simulink model "pruebas_filtro_lcl"  (R2024a)
settings: Solver=VariableStepAuto  StartTime=0.0  StopTime=5  RelTol=1e-3
libraries: spsThreePhaseSeriesRLCBranchLib x3, spsGroundLib x2, spsDCVoltageSourceLib x1, spsTwoLevelConverterLib x1, spsSVPWMGenerator2LevelLib x1, spsThreePhaseVIMeasurementLib x1, spsThreePhaseProgrammableVoltageSourceLib x1, sps_lib x1
settings Model: SimulationMode=accelerator  Creator=sebar  LastModifiedBy=sebar

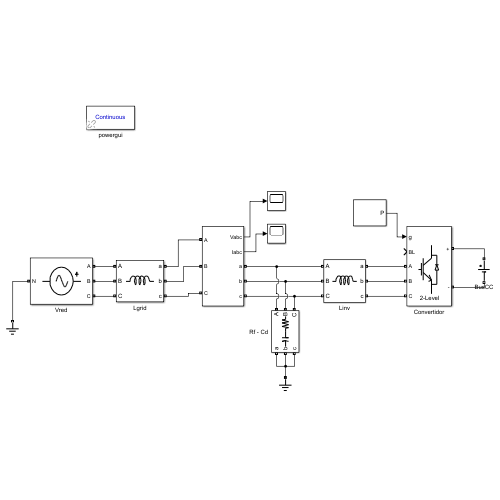
[thumbnail: Simulink's stored preview of the top-level diagram]
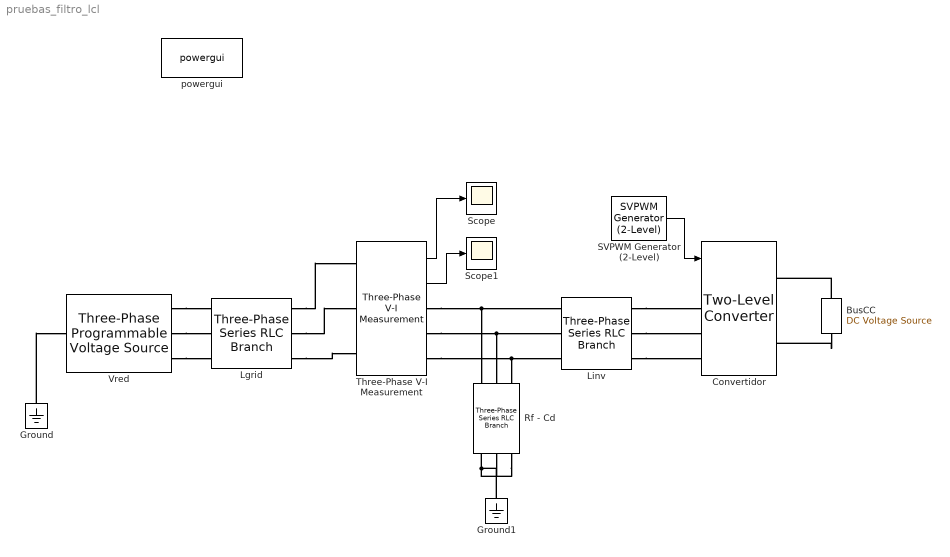
== system pruebas_filtro_lcl ==
  BusCC : spsDCVoltageSourceLib/DC Voltage Source  Amplitude=400  Measurements=None
  Convertidor : spsTwoLevelConverterLib/Two-Level Converter  ModelType=Switching devices  Ron=1e-3  Rs=1e6  Cs=inf  Vforward=[0,0]  Ron_Diode=1e-3  Rs_Diode=1e6  Cs_Diode=inf  Vf_Diode=1e-3  Rs_CurrentSource=inf  Ron_ACsource=1e-3
      settings: LibrarySourceBlock=sps_lib/Power Electronics/Two-Level Converter
  Ground : spsGroundLib/Ground  LConnTagsString=a
  Ground1 : spsGroundLib/Ground  LConnTagsString=a
  Lgrid : spsThreePhaseSeriesRLCBranchLib/Three-Phase Series RLC Branch  LConnTagsString=A|B|C  RConnTagsString=A|B|C  BranchType=L  Resistance=1  Inductance=273e-6  Capacitance=1e-6  Measurements=None
  Linv : spsThreePhaseSeriesRLCBranchLib/Three-Phase Series RLC Branch  LConnTagsString=A|B|C  RConnTagsString=A|B|C  BranchType=L  Resistance=1  Inductance=263e-6  Capacitance=1e-6  Measurements=None
  Rf - Cd : spsThreePhaseSeriesRLCBranchLib/Three-Phase Series RLC Branch  LConnTagsString=A|B|C  RConnTagsString=A|B|C  BranchType=RC  Resistance=0.89  Inductance=1e-3  Capacitance=18.5e-6  Measurements=None
  SVPWM Generator (2-Level) : spsSVPWMGenerator2LevelLib/SVPWM Generator (2-Level)  InputType=Internally generated  SwitchingPattern=Pattern #1  Fc=10000  ParUref=[0.796084166 0 50]  Ts=0
  Scope : Scope
  Scope1 : Scope
  Three-Phase V-I Measurement : spsThreePhaseVIMeasurementLib/Three-Phase V-I Measurement  VoltageMeasurement=phase-to-ground  SetLabelV=off  LabelV=Vabc  Vpu=off  VpuLL=off  CurrentMeasurement=yes  SetLabelI=off  LabelI=Iabc  Ipu=off  Pbase=100e6  Vbase=500e3  OutputType=Complex  PhasorSimulation=off  PSBequivalent=0
  Vred : spsThreePhaseProgrammableVoltageSourceLib/Three-Phase Programmable Voltage Source  PositiveSequence="[130*sqrt(3)  0 50]"  VariationEntity=None  VariationType=Table of time-amplitude pairs  VariationTypeAlt=Step  VariationStep=0.5  VariationRate=10  VariationMagnitude=0.3  VariationFrequency=2  VariationTiming=[1 2]  VariationPhaseA=off  Amplitudes=[1 0.8 1.2 1.0]  TimeValues=[0 0.1 0.15 0.2]  HarmonicGeneration=off  HarmonicA=[3 0.2 -25 0]  HarmonicB=[2 0.15 35 2]  Timing="[0.05  3]"  BusType=swing  Pref=0  Qref=0  Qmin=-inf  Qmax=inf
  powergui : sps_lib/powergui  Priority=1  SimulationMode=Continuous  SampleTime=50e-6  frequency=60  Iterations=50  frequencyindice=50  Pbase=100e6  ErrMax=1e-4  UnitsV=kV  UnitsW=MW  buscounter=0  FunctionMessages=off  echomessages=off  EnableUseOfTLC=off  CurrentSourceSwitches=off  DisableSnubberDevices=off  DisableRonSwitches=off  DisableVfSwitches=off  DisplayEquations=on  AutomaticDiscreteSolvers=off  SolverType=Tustin/Backward Euler (TBE)  Interpol=off  ExternalGateDelay=off  methode=off  Ts=100  x0status=steady  SPID=on  SwTol=0  HookPort=off  NonlinearTolerance=1e-4  nMaxIteration=100  ContinueOnMaxIteration=off  RestoreLinks=warning  ResistiveCurrentMeasurement=off  Frange=[0:2:500]  Ylog=off  Xlog=on  ShowGrid=off  save=off  variable=ZData  structure=0  ZoomFFT=off  StartTime=0.0  cycles=1  DisplayStyle=1  fundamental=60  FreqAxis=off  MaxFrequency=1000  frequencyindicesteady=1  RmsSteady=1  display=off
  wires:
  SVPWM Generator (2-Level)/1 -> Convertidor/1
  Three-Phase V-I Measurement/2 -> Scope1/1
  Three-Phase V-I Measurement/1 -> Scope/1
  connections:
  BusCC/RConn1 -- Convertidor/RConn1
  BusCC/LConn1 -- Convertidor/RConn2
  Vred/RConn1 -- Lgrid/LConn1
  Vred/RConn2 -- Lgrid/LConn2
  Vred/RConn3 -- Lgrid/LConn3
  Lgrid/RConn1 -- Three-Phase V-I Measurement/LConn1
  Lgrid/RConn2 -- Three-Phase V-I Measurement/LConn2
  Lgrid/RConn3 -- Three-Phase V-I Measurement/LConn3
  Three-Phase V-I Measurement/RConn1 -- Linv/LConn1 -- Rf - Cd/LConn1
  Three-Phase V-I Measurement/RConn2 -- Rf - Cd/LConn2 -- Linv/LConn2
  Three-Phase V-I Measurement/RConn3 -- Linv/LConn3 -- Rf - Cd/LConn3
  Linv/RConn1 -- Convertidor/LConn1
  Linv/RConn2 -- Convertidor/LConn2
  Linv/RConn3 -- Convertidor/LConn3
  Ground/LConn1 -- Vred/LConn1
  Rf - Cd/RConn1 -- Ground1/LConn1 -- Rf - Cd/RConn3 -- Rf - Cd/RConn2
